simulink model "model_robot"  (R2024a)
settings: Solver=ode45  StartTime=0  StopTime=.5  FixedStep=0.01  RelTol=1e-3
undefined symbols (not defined in the file or in its folder): A, B, b10, b20, f0, g0, gamma0, m0, r_max, r_min, theta_max, theta_min, x10, x20, x30, x40
settings Model: Creator=brzan  LastModifiedBy=brzan

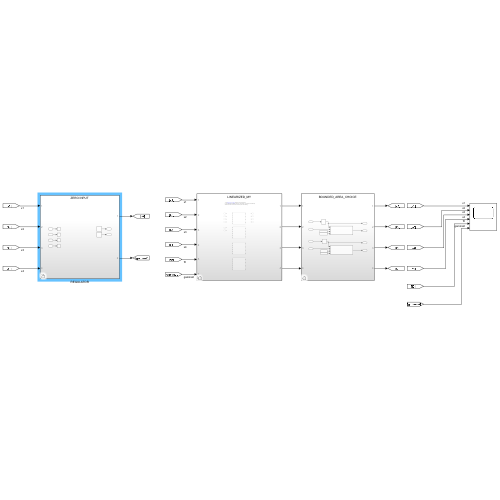
[thumbnail: Simulink's stored preview of the top-level diagram]
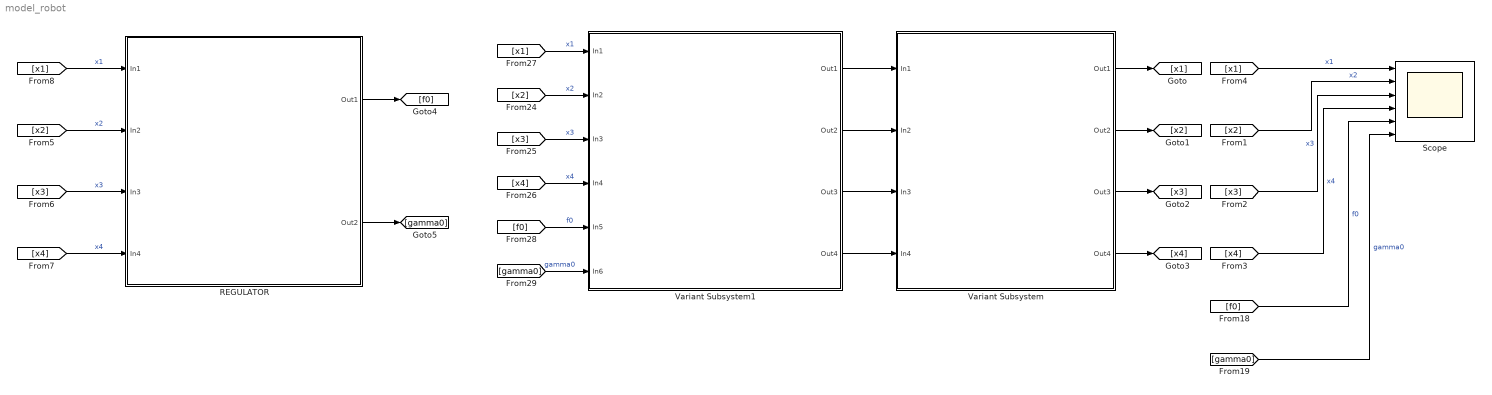
== system model_robot ==
  REGULATOR : Subsystem  Variant=on
  Scope : Scope  NumInputPorts=6
  Variant Subsystem : Subsystem  Variant=on
  Variant Subsystem1 : Subsystem  Variant=on
  wires:
  [x4] -> Scope/4  "x4"
  [x3] -> Scope/3  "x3"
  [x2] -> Scope/2  "x2"
  [x1] -> Scope/1  "x1"
  [f0] -> Scope/5  "f0"
  [gamma0] -> Scope/6  "gamma0"
  Variant Subsystem1/1(Out1) -> Variant Subsystem/1(In1)
  Variant Subsystem1/2(Out2) -> Variant Subsystem/2(In2)
  Variant Subsystem1/3(Out3) -> Variant Subsystem/3(In3)
  Variant Subsystem1/4(Out4) -> Variant Subsystem/4(In4)
  Variant Subsystem/1(Out1) -> [x1]
  Variant Subsystem/2(Out2) -> [x2]
  Variant Subsystem/3(Out3) -> [x3]
  Variant Subsystem/4(Out4) -> [x4]
  [x4] -> Variant Subsystem1/4(In4)  "x4"
  [x3] -> Variant Subsystem1/3(In3)  "x3"
  [x2] -> Variant Subsystem1/2(In2)  "x2"
  [x1] -> Variant Subsystem1/1(In1)  "x1"
  [f0] -> Variant Subsystem1/5(In5)  "f0"
  [gamma0] -> Variant Subsystem1/6(In6)  "gamma0"
  REGULATOR/2(Out2) -> [gamma0]
  REGULATOR/1(Out1) -> [f0]
  [x1] -> REGULATOR/1(In1)  "x1"
  [x2] -> REGULATOR/2(In2)  "x2"
  [x3] -> REGULATOR/3(In3)  "x3"
  [x4] -> REGULATOR/4(In4)  "x4"

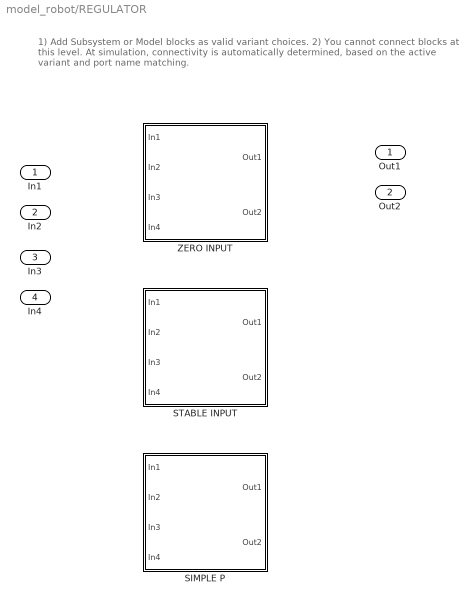
== system model_robot/REGULATOR ==
  note: 1) Add Subsystem or Model blocks as valid variant choices.
      | 2) You cannot connect blocks at this level. At simulation, connectivity is automatically
      | determined, based on the active variant and port name matching.
  In1 : Inport
  In2 : Inport  Port=2
  In3 : Inport  Port=3
  In4 : Inport  Port=4
  SIMPLE P : Subsystem  VariantControl="REGULATOR_CHOICE == \"SIMPLE\""
  STABLE INPUT : Subsystem  VariantControl="REGULATOR_CHOICE == \"STABLE_INPUT\""
  ZERO INPUT : Subsystem  VariantControl="REGULATOR_CHOICE == \"ZERO_INPUT\""
  Out1 : Outport
  Out2 : Outport  Port=2

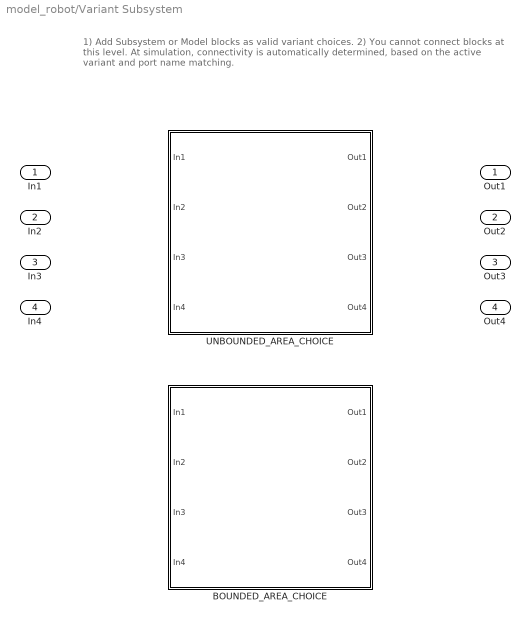
== system model_robot/Variant Subsystem ==
  note: 1) Add Subsystem or Model blocks as valid variant choices.
      | 2) You cannot connect blocks at this level. At simulation, connectivity is automatically
      | determined, based on the active variant and port name matching.
  In1 : Inport
  In2 : Inport  Port=2
  In3 : Inport  Port=3
  In4 : Inport  Port=4
  BOUNDED_AREA_CHOICE : Subsystem  VariantControl="BOUNDARY_CHOICE == \"BOUNDED\""
  UNBOUNDED_AREA_CHOICE : Subsystem  VariantControl="BOUNDARY_CHOICE == \"UNBOUNDED\""
  Out1 : Outport
  Out2 : Outport  Port=2
  Out3 : Outport  Port=3
  Out4 : Outport  Port=4

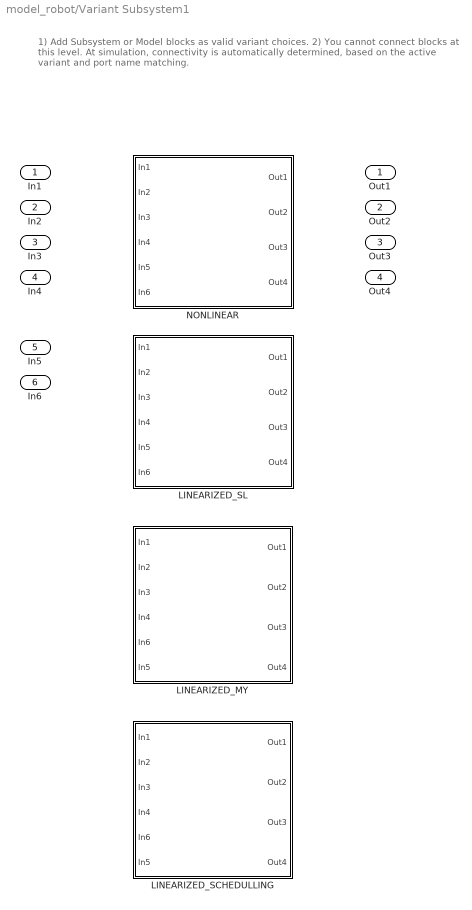
== system model_robot/Variant Subsystem1 ==
  note: 1) Add Subsystem or Model blocks as valid variant choices.
      | 2) You cannot connect blocks at this level. At simulation, connectivity is automatically
      | determined, based on the active variant and port name matching.
  In1 : Inport
  In2 : Inport  Port=2
  In3 : Inport  Port=3
  In4 : Inport  Port=4
  In5 : Inport  Port=5
  In6 : Inport  Port=6
  LINEARIZED_MY : Subsystem  VariantControl="MODEL_CHOICE == \"LINEARIZED_MY\""
  LINEARIZED_SCHEDULLING : Subsystem  VariantControl="MODEL_CHOICE == \"LINEARIZED_MY\""
  LINEARIZED_SL : Subsystem  VariantControl="MODEL_CHOICE == \"LINEARIZED_SL\""
  NONLINEAR : Subsystem  VariantControl="MODEL_CHOICE == \"NONLINEAR\""
  Out1 : Outport
  Out2 : Outport  Port=2
  Out3 : Outport  Port=3
  Out4 : Outport  Port=4

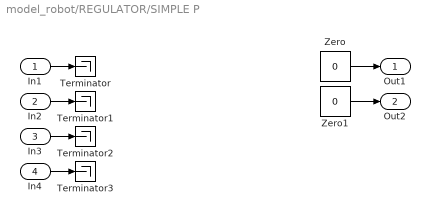
== system model_robot/REGULATOR/SIMPLE P ==
  In1 : Inport
  In2 : Inport  Port=2
  In3 : Inport  Port=3
  In4 : Inport  Port=4
  Terminator{,1..3} (4 alike) : Terminator
  Zero : Constant  Value=0  OutDataTypeStr=Inherit: Inherit via back propagation
  Zero1 : Constant  Value=0  OutDataTypeStr=Inherit: Inherit via back propagation
  Out1 : Outport
  Out2 : Outport  Port=2
  wires:
  In1/1 -> Terminator/1
  In2/1 -> Terminator1/1
  In3/1 -> Terminator2/1
  In4/1 -> Terminator3/1
  Zero/1 -> Out1/1
  Zero1/1 -> Out2/1

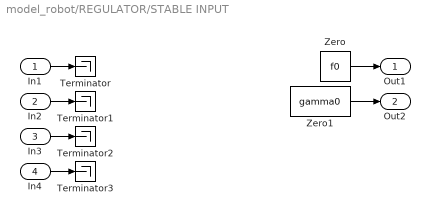
== system model_robot/REGULATOR/STABLE INPUT ==
  In1 : Inport
  In2 : Inport  Port=2
  In3 : Inport  Port=3
  In4 : Inport  Port=4
  Terminator{,1..3} (4 alike) : Terminator
  Zero : Constant  Value=f0  OutDataTypeStr=Inherit: Inherit via back propagation
  Zero1 : Constant  Value=gamma0  OutDataTypeStr=Inherit: Inherit via back propagation
  Out1 : Outport
  Out2 : Outport  Port=2
  wires:
  In1/1 -> Terminator/1
  In2/1 -> Terminator1/1
  In3/1 -> Terminator2/1
  In4/1 -> Terminator3/1
  Zero/1 -> Out1/1
  Zero1/1 -> Out2/1

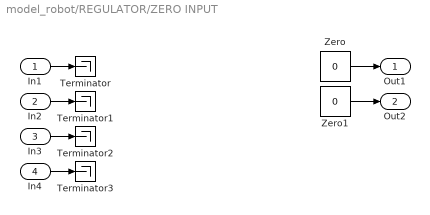
== system model_robot/REGULATOR/ZERO INPUT ==
  In1 : Inport
  In2 : Inport  Port=2
  In3 : Inport  Port=3
  In4 : Inport  Port=4
  Terminator{,1..3} (4 alike) : Terminator
  Zero : Constant  Value=0  OutDataTypeStr=Inherit: Inherit via back propagation
  Zero1 : Constant  Value=0  OutDataTypeStr=Inherit: Inherit via back propagation
  Out1 : Outport
  Out2 : Outport  Port=2
  wires:
  In1/1 -> Terminator/1
  In2/1 -> Terminator1/1
  In3/1 -> Terminator2/1
  In4/1 -> Terminator3/1
  Zero/1 -> Out1/1
  Zero1/1 -> Out2/1

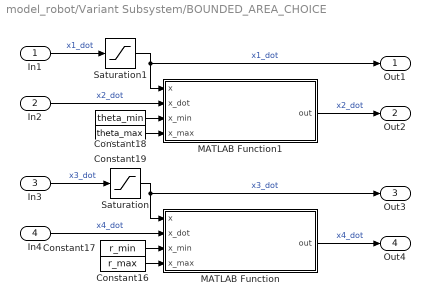
== system model_robot/Variant Subsystem/BOUNDED_AREA_CHOICE ==
  In1 : Inport
  In2 : Inport  Port=2
  In3 : Inport  Port=3
  In4 : Inport  Port=4
  Constant16 : Constant  Value=r_max
  Constant17 : Constant  Value=r_min
  Constant18 : Constant  Value=theta_min
  Constant19 : Constant  Value=theta_max
  MATLAB Function : MATLAB Function  TreatAsAtomicUnit=on
  MATLAB Function1 : MATLAB Function  TreatAsAtomicUnit=on
  Saturation : Saturate  UpperLimit=r_max  LowerLimit=r_min
  Saturation1 : Saturate  UpperLimit=theta_max  LowerLimit=theta_min
  Out1 : Outport
  Out2 : Outport  Port=2
  Out3 : Outport  Port=3
  Out4 : Outport  Port=4
  wires:
  In3/1 -> Saturation/1  "x3_dot"
  Constant18/1 -> MATLAB Function1/3(x_min)
  In1/1 -> Saturation1/1  "x1_dot"
  Saturation1/1 -> Out1/1, MATLAB Function1/1(x)  "x1_dot"
  Saturation/1 -> Out3/1, MATLAB Function/1(x)  "x3_dot"
  Constant17/1 -> MATLAB Function/3(x_min)
  Constant16/1 -> MATLAB Function/4(x_max)
  Constant19/1 -> MATLAB Function1/4(x_max)
  MATLAB Function1/1(out) -> Out2/1  "x2_dot"
  In2/1 -> MATLAB Function1/2(x_dot)  "x2_dot"
  In4/1 -> MATLAB Function/2(x_dot)  "x4_dot"
  MATLAB Function/1(out) -> Out4/1  "x4_dot"

== system model_robot/Variant Subsystem/UNBOUNDED_AREA_CHOICE ==
  In1 : Inport
  In2 : Inport  Port=2
  In3 : Inport  Port=3
  In4 : Inport  Port=4
  Out1 : Outport
  Out2 : Outport  Port=2
  Out3 : Outport  Port=3
  Out4 : Outport  Port=4
  wires:
  In1/1 -> Out1/1
  In2/1 -> Out2/1
  In3/1 -> Out3/1
  In4/1 -> Out4/1

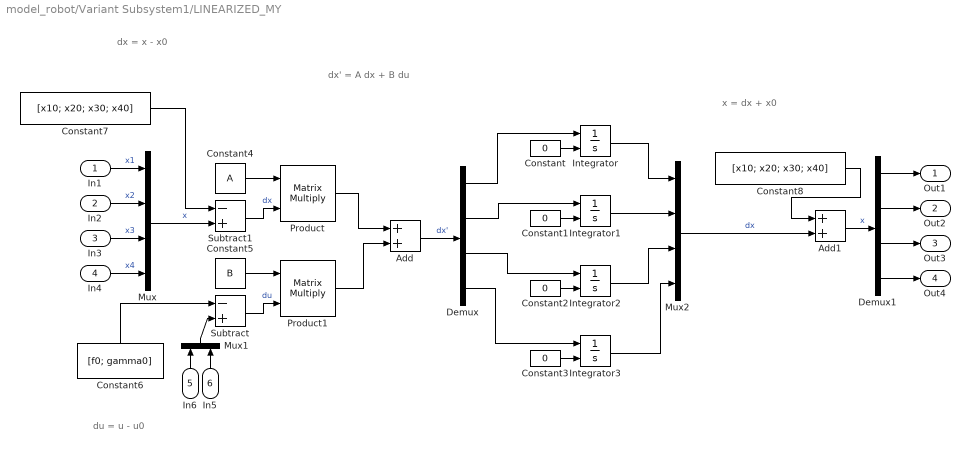
== system model_robot/Variant Subsystem1/LINEARIZED_MY ==
  note: dx' = A dx + B du
  note: x = dx + x0
  note: dx = x - x0
  note: du = u - u0
  In1 : Inport
  In2 : Inport  Port=2
  In3 : Inport  Port=3
  In4 : Inport  Port=4
  In6 : Inport  Port=5
  In5 : Inport  Port=6
  Add : Sum
  Add1 : Sum
  Constant{,1..3} (4 alike) : Constant  Value=0
  Constant4 : Constant  Value=A  VectorParams1D=off
  Constant5 : Constant  Value=B  VectorParams1D=off
  Constant6 : Constant  Value=[f0; gamma0]  VectorParams1D=off
  Constant7 : Constant  Value=[x10; x20; x30; x40]  VectorParams1D=off
  Constant8 : Constant  Value=[x10; x20; x30; x40]  VectorParams1D=off
  Demux : Demux
  Demux1 : Demux
  Integrator{,1..3} (4 alike) : Integrator  InitialConditionSource=external
  Mux : Mux
  Mux1 : Mux  Inputs=2
  Mux2 : Mux
  Product : Product  Multiplication=Matrix(*)
  Product1 : Product  Multiplication=Matrix(*)
  Subtract : Sum  Inputs=-+
  Subtract1 : Sum  Inputs=-+
  Out1 : Outport
  Out2 : Outport  Port=2
  Out3 : Outport  Port=3
  Out4 : Outport  Port=4
  wires:
  In4/1 -> Mux/4  "x4"
  In3/1 -> Mux/3  "x3"
  In2/1 -> Mux/2  "x2"
  In1/1 -> Mux/1  "x1"
  Integrator3/1 -> Mux2/4
  Integrator/1 -> Mux2/1
  Demux/4 -> Integrator3/1
  Constant3/1 -> Integrator3/2
  Demux/1 -> Integrator/1
  Demux/3 -> Integrator2/1
  Constant1/1 -> Integrator1/2
  Integrator1/1 -> Mux2/2
  Constant/1 -> Integrator/2
  Integrator2/1 -> Mux2/3
  Constant2/1 -> Integrator2/2
  Demux/2 -> Integrator1/1
  Constant4/1 -> Product/1
  Mux/1 -> Subtract1/2  "x"
  Constant5/1 -> Product1/1
  Product/1 -> Add/1
  Product1/1 -> Add/2
  Add/1 -> Demux/1  "dx'"
  In5/1 -> Mux1/2
  In6/1 -> Mux1/1
  Mux1/1 -> Subtract/2
  Subtract/1 -> Product1/2  "du"
  Constant6/1 -> Subtract/1
  Subtract1/1 -> Product/2  "dx"
  Constant7/1 -> Subtract1/1
  Demux1/1 -> Out1/1
  Demux1/2 -> Out2/1
  Demux1/3 -> Out3/1
  Demux1/4 -> Out4/1
  Add1/1 -> Demux1/1  "x"
  Constant8/1 -> Add1/1
  Mux2/1 -> Add1/2  "dx"

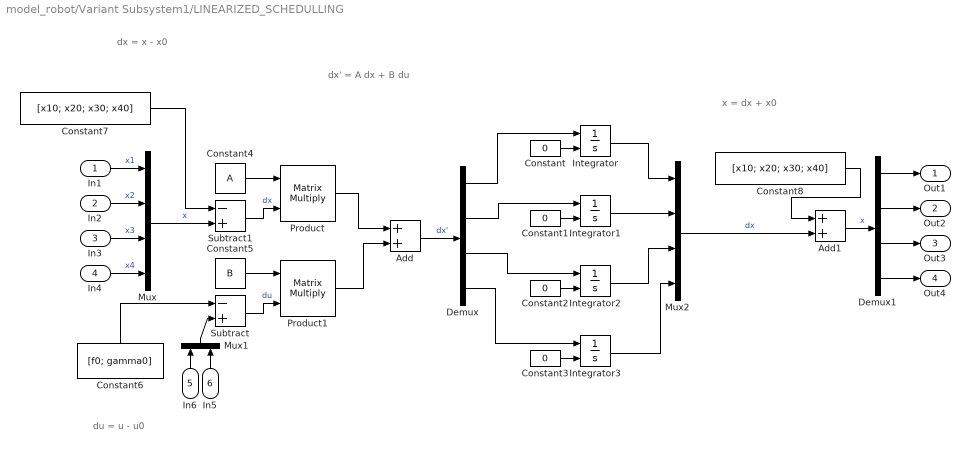
== system model_robot/Variant Subsystem1/LINEARIZED_SCHEDULLING ==
  note: dx' = A dx + B du
  note: x = dx + x0
  note: dx = x - x0
  note: du = u - u0
  In1 : Inport
  In2 : Inport  Port=2
  In3 : Inport  Port=3
  In4 : Inport  Port=4
  In6 : Inport  Port=5
  In5 : Inport  Port=6
  Add : Sum
  Add1 : Sum
  Constant{,1..3} (4 alike) : Constant  Value=0
  Constant4 : Constant  Value=A  VectorParams1D=off
  Constant5 : Constant  Value=B  VectorParams1D=off
  Constant6 : Constant  Value=[f0; gamma0]  VectorParams1D=off
  Constant7 : Constant  Value=[x10; x20; x30; x40]  VectorParams1D=off
  Constant8 : Constant  Value=[x10; x20; x30; x40]  VectorParams1D=off
  Demux : Demux
  Demux1 : Demux
  Integrator{,1..3} (4 alike) : Integrator  InitialConditionSource=external
  Mux : Mux
  Mux1 : Mux  Inputs=2
  Mux2 : Mux
  Product : Product  Multiplication=Matrix(*)
  Product1 : Product  Multiplication=Matrix(*)
  Subtract : Sum  Inputs=-+
  Subtract1 : Sum  Inputs=-+
  Out1 : Outport
  Out2 : Outport  Port=2
  Out3 : Outport  Port=3
  Out4 : Outport  Port=4
  wires:
  In4/1 -> Mux/4  "x4"
  In3/1 -> Mux/3  "x3"
  In2/1 -> Mux/2  "x2"
  In1/1 -> Mux/1  "x1"
  Integrator3/1 -> Mux2/4
  Integrator/1 -> Mux2/1
  Demux/4 -> Integrator3/1
  Constant3/1 -> Integrator3/2
  Demux/1 -> Integrator/1
  Demux/3 -> Integrator2/1
  Constant1/1 -> Integrator1/2
  Integrator1/1 -> Mux2/2
  Constant/1 -> Integrator/2
  Integrator2/1 -> Mux2/3
  Constant2/1 -> Integrator2/2
  Demux/2 -> Integrator1/1
  Constant4/1 -> Product/1
  Mux/1 -> Subtract1/2  "x"
  Constant5/1 -> Product1/1
  Product/1 -> Add/1
  Product1/1 -> Add/2
  Add/1 -> Demux/1  "dx'"
  In5/1 -> Mux1/2
  In6/1 -> Mux1/1
  Mux1/1 -> Subtract/2
  Subtract/1 -> Product1/2  "du"
  Constant6/1 -> Subtract/1
  Subtract1/1 -> Product/2  "dx"
  Constant7/1 -> Subtract1/1
  Demux1/1 -> Out1/1
  Demux1/2 -> Out2/1
  Demux1/3 -> Out3/1
  Demux1/4 -> Out4/1
  Add1/1 -> Demux1/1  "x"
  Constant8/1 -> Add1/1
  Mux2/1 -> Add1/2  "dx"

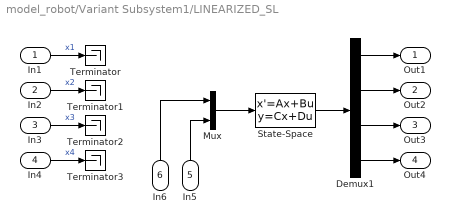
== system model_robot/Variant Subsystem1/LINEARIZED_SL ==
  In1 : Inport
  In2 : Inport  Port=2
  In3 : Inport  Port=3
  In4 : Inport  Port=4
  In5 : Inport  Port=5
  In6 : Inport  Port=6
  Demux1 : Demux
  Mux : Mux  Inputs=2
  State-Space : StateSpace  A=A  B=B  C=eye(4)  D=zeros([4 2])  InitialCondition=[x10 x20 x30 x40]
  Terminator{,1..3} (4 alike) : Terminator
  Out1 : Outport
  Out2 : Outport  Port=2
  Out3 : Outport  Port=3
  Out4 : Outport  Port=4
  wires:
  Mux/1 -> State-Space/1
  In4/1 -> Terminator3/1  "x4"
  In3/1 -> Terminator2/1  "x3"
  In2/1 -> Terminator1/1  "x2"
  In1/1 -> Terminator/1  "x1"
  In6/1 -> Mux/1
  In5/1 -> Mux/2
  Demux1/1 -> Out1/1
  Demux1/2 -> Out2/1
  Demux1/3 -> Out3/1
  Demux1/4 -> Out4/1
  State-Space/1 -> Demux1/1

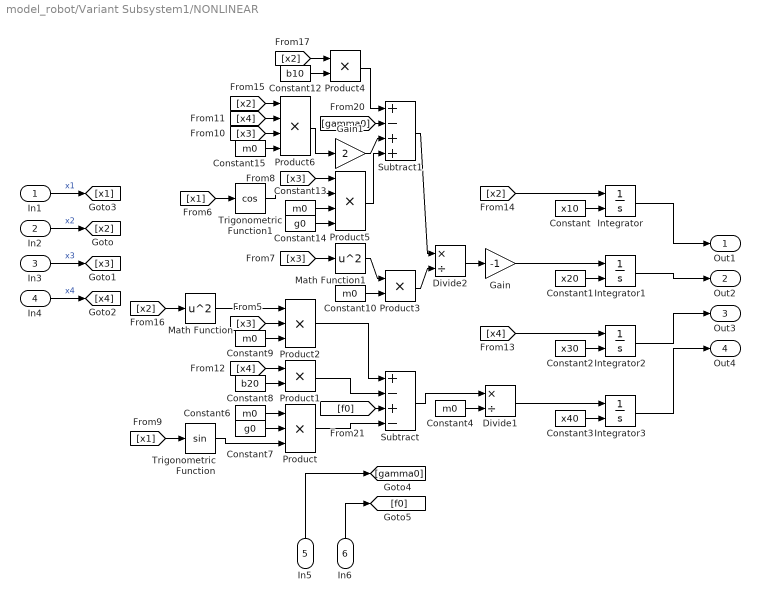
== system model_robot/Variant Subsystem1/NONLINEAR ==
  In1 : Inport
  In2 : Inport  Port=2
  In3 : Inport  Port=3
  In4 : Inport  Port=4
  In5 : Inport  Port=5
  In6 : Inport  Port=6
  Constant : Constant  Value=x10
  Constant1 : Constant  Value=x20
  Constant{4,6,9..10,13,15} (6 alike) : Constant  Value=m0
  Constant12 : Constant  Value=b10
  Constant14 : Constant  Value=g0
  Constant2 : Constant  Value=x30
  Constant3 : Constant  Value=x40
  Constant7 : Constant  Value=g0
  Constant8 : Constant  Value=b20
  Divide1 : Product  Inputs=*/
  Divide2 : Product  Inputs=*/
  Gain : Gain  Gain=-1
  Gain1 : Gain  Gain=2
  Integrator{,1..3} (4 alike) : Integrator  InitialConditionSource=external
  Math Function : Math  Operator=square
  Math Function1 : Math  Operator=square
  Product : Product  Inputs=3
  Product1 : Product
  Product2 : Product  Inputs=3
  Product3 : Product
  Product4 : Product
  Product5 : Product  Inputs=4
  Product6 : Product  Inputs=4
  Subtract : Sum  Inputs=+-+-
  Subtract1 : Sum  Inputs=+-++
  Trigonometric Function : Trigonometry
  Trigonometric Function1 : Trigonometry  Operator=cos
  Out1 : Outport
  Out2 : Outport  Port=2
  Out3 : Outport  Port=3
  Out4 : Outport  Port=4
  wires:
  Constant7/1 -> Product/2
  Product/1 -> Subtract/4
  Subtract1/1 -> Divide2/1
  Product2/1 -> Subtract/1
  Constant15/1 -> Product6/4
  [f0] -> Subtract/3
  Constant9/1 -> Product2/3
  [x3] -> Product2/2
  [gamma0] -> Subtract1/2
  Constant12/1 -> Product4/2
  Product1/1 -> Subtract/2
  Math Function1/1 -> Product3/1
  Constant10/1 -> Product3/2
  Divide2/1 -> Gain/1
  Subtract/1 -> Divide1/1
  Product3/1 -> Divide2/2
  Gain1/1 -> Subtract1/3
  [x2] -> Product4/1
  Constant6/1 -> Product/1
  Constant13/1 -> Product5/3
  [x1] -> Trigonometric Function/1
  Product5/1 -> Subtract1/4
  Product4/1 -> Subtract1/1
  Math Function/1 -> Product2/1
  [x4] -> Product6/2
  Constant4/1 -> Divide1/2
  Trigonometric Function/1 -> Product/3
  [x4] -> Product1/1
  Product6/1 -> Gain1/1
  [x2] -> Math Function/1
  [x3] -> Product5/1
  Constant8/1 -> Product1/2
  [x2] -> Product6/1
  Trigonometric Function1/1 -> Product5/2
  [x1] -> Trigonometric Function1/1
  [x3] -> Math Function1/1
  Constant14/1 -> Product5/4
  [x3] -> Product6/3
  In2/1 -> [x2]  "x2"
  In3/1 -> [x3]  "x3"
  In4/1 -> [x4]  "x4"
  In1/1 -> [x1]  "x1"
  In6/1 -> [f0]
  In5/1 -> [gamma0]
  Constant/1 -> Integrator/2
  Constant2/1 -> Integrator2/2
  Gain/1 -> Integrator1/1
  [x4] -> Integrator2/1
  [x2] -> Integrator/1
  Divide1/1 -> Integrator3/1
  Constant1/1 -> Integrator1/2
  Constant3/1 -> Integrator3/2
  Integrator/1 -> Out1/1
  Integrator1/1 -> Out2/1
  Integrator2/1 -> Out3/1
  Integrator3/1 -> Out4/1

== matlab function model_robot/Variant Subsystem/BOUNDED_AREA_CHOICE/MATLAB Function1 ==
  data: x input; out output; x_dot input; x_min input; x_max input
function out = saturate_velocity(x, x_dot, x_min, x_max)
    if (x >= x_max && x_dot > 0) || (x <= x_min && x_dot < 0)
        out = 0;
    else
        out = x_dot;
    end
end

== matlab function model_robot/Variant Subsystem/BOUNDED_AREA_CHOICE/MATLAB Function ==
  data: x input; out output; x_dot input; x_min input; x_max input
function out = saturate_velocity(x, x_dot, x_min, x_max)
    if (x >= x_max && x_dot > 0) || (x <= x_min && x_dot < 0)
        out = 0;
    else
        out = x_dot;
    end
end
